simulink model "BilateralFilterHDLExample"  (R2019b)
settings: Solver=FixedStepDiscrete  StartTime=0.0  StopTime=9  RelTol=1e-3
undefined symbols (not defined in the file): gray, Rec, SDTV
libraries: visionhdlio x2, dspvision x1, visionhdlutilities x1, visionhdlfilter x1, visionhdlconversions x1, visionhdlanalysis x1
settings Model: DataTypeOverride=Off  SimulationMode=accelerator  Creator=The MathWorks, Inc.  LastModifiedBy=Bilal
settings SolverCC: MinimalZcImpactIntegration=on
settings DataIOCC: SaveOutput=off  SaveTime=off  ReturnWorkspaceOutputs=off
settings OptimizationCC: BlockReduction=off  ConditionallyExecuteInputs=off  DefaultParameterBehavior=Inlined
settings DebuggingCC: AlgebraicLoopMsg=error  SingleTaskRateTransMsg=error  ArithmeticOperatorsInVariantConditions=warning
settings HardwareCC: ProdBitPerPointer=32  ProdBitPerSizeT=32  ProdBitPerPtrDiffT=32  ProdLargestAtomicFloat=None  ProdIntDivRoundTo=Undefined  ProdEndianess=Unspecified  ProdWordSize=32  ProdHWDeviceType=ASIC/FPGA->ASIC/FPGA  ProdEqTarget=off
settings SFSimCC: SimUseLocalCustomCode=off  CustomCodeUndefinedFunction=UseInterfaceOnly
settings RTWCC: RTWUseLocalCustomCode=off
settings CodeAppCC: StateflowObjectComments=on

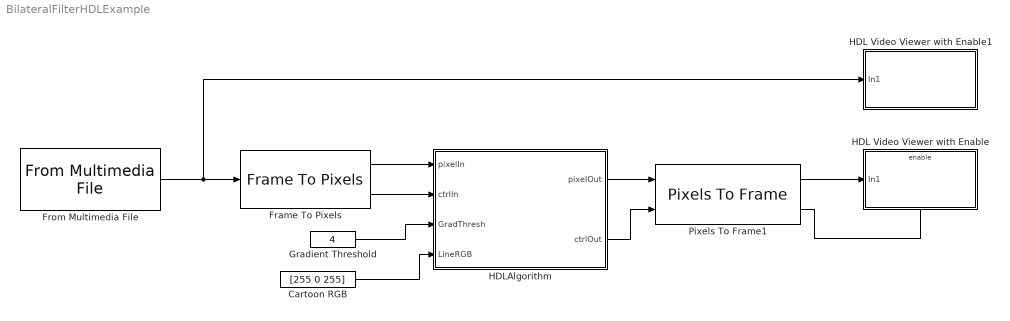
== system BilateralFilterHDLExample ==
  Cartoon RGB : Constant  Value=[255 0 255]  OutDataTypeStr=Inherit: Inherit via back propagation  SampleTime=-1
  Frame To Pixels : visionhdlio/Frame To Pixels  NumComponents=3  NumPixels=1  VideoFormat=Custom  ActivePixelsPerLine=320  ActiveVideoLines=180  TotalPixelsPerLine=400  TotalVideoLines=240  StartingActiveLine=6  FrontPorch=10  SampleTime=0
      settings: SourceProductName=Vision HDL Toolbox  SourceProductBaseCode=VT
  From Multimedia File : dspvision/From Multimedia File  inputFilename=potholes2.avi  readRange=[1 Inf]  loop=on  numPlays=inf  outputStreams=Video only  videoDataType=uint8  audioDataType=int16  inheritSampleTime=on  userDefinedSampleTime=1/30  noAudioOutput=off  isIntensityVideo=off  fourcc=RGB  colorVideoFormat=One multidimensional signal  outputEOF=off  dataOrg=Column-major  audioFrameSize=1024  computeAudioFrameSize=off  outSamplingMode=Sample based
      settings: SourceProductName=DSP System Toolbox  SourceProductBaseCode=DS
  Gradient Threshold : Constant  Value=4  OutDataTypeStr=uint8  SampleTime=-1
  HDL Video Viewer with Enable : Subsystem
  HDL Video Viewer with Enable1 : Subsystem
  HDLAlgorithm : Subsystem
  Pixels To Frame1 : visionhdlio/Pixels To Frame  NumComponents=3  NumPixels=1  VideoFormat=Custom  ActivePixelsPerLine=320  ActiveVideoLines=180  TotalPixelsPerLine=400  TotalVideoLines=240
      settings: SourceProductName=Vision HDL Toolbox  SourceProductBaseCode=VT
  wires:
  Frame To Pixels/1 -> HDLAlgorithm/1(pixelIn)
  HDLAlgorithm/2(ctrlOut) -> Pixels To Frame1/2
  HDLAlgorithm/1(pixelOut) -> Pixels To Frame1/1
  Frame To Pixels/2 -> HDLAlgorithm/2(ctrlIn)
  Pixels To Frame1/1 -> HDL Video Viewer with Enable/1(In1)
  Pixels To Frame1/2 -> HDL Video Viewer with Enable/Enable
  From Multimedia File/1 -> HDL Video Viewer with Enable1/1(In1), Frame To Pixels/1
  Gradient Threshold/1 -> HDLAlgorithm/3(GradThresh)
  Cartoon RGB/1 -> HDLAlgorithm/4(LineRGB)

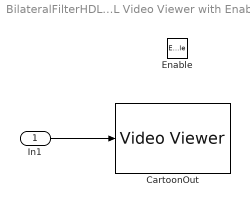
== system BilateralFilterHDLExample/HDL Video Viewer with Enable ==
  In1 : Inport
  Enable : EnablePort
  CartoonOut : VideoViewer  colormapValue=gray(256)  FigPos=[420 351 320 243]
  wires:
  In1/1 -> CartoonOut/1

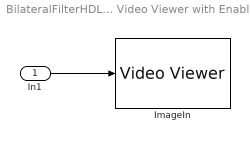
== system BilateralFilterHDLExample/HDL Video Viewer with Enable1 ==
  In1 : Inport
  ImageIn : VideoViewer  colormapValue=gray(256)  FigPos=[249 353 321 244]
  wires:
  In1/1 -> ImageIn/1

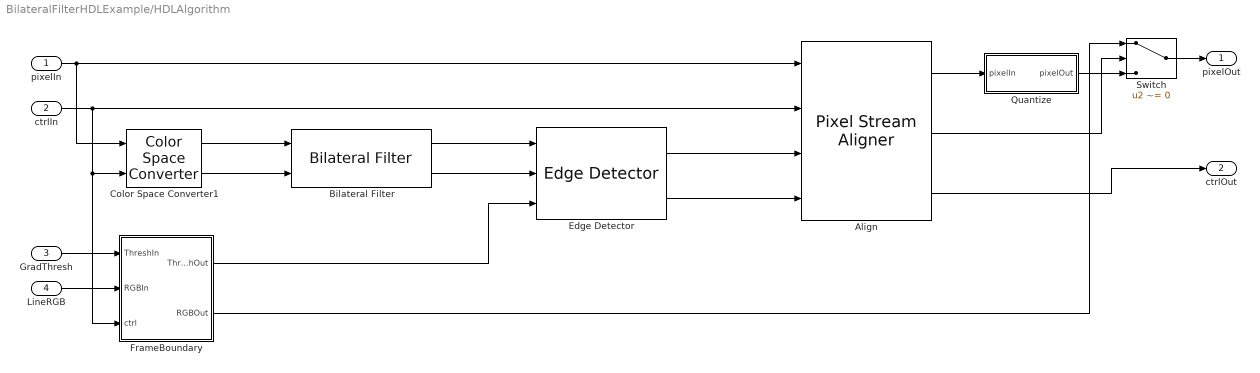
== system BilateralFilterHDLExample/HDLAlgorithm ==
  pixelIn : Inport
  ctrlIn : Inport  Port=2
  GradThresh : Inport  Port=3
  LineRGB : Inport  Port=4
  Align : visionhdlutilities/Pixel Stream Aligner  LineBufferSize=2048  MaximumNumberOfLines=10  SimulateUsing=Code generation
      settings: SourceProductName=Vision HDL Toolbox  SourceProductBaseCode=VT
  Bilateral Filter : visionhdlfilter/Bilateral Filter  NeighborhoodSize=9x9  SpatialStdDev=3  IntensityStdDev=0.75  PaddingMethod=Replicate  PaddingValue=0  LineBufferSize=2048  SimulateUsing=Code generation  CoefficientsDataTypeStr=fixdt(0,22,22)  roundingMode=Nearest  overflowMode=on  OutputDataTypeStr=fixdt(0,8,0)  OutputMin=[]  OutputMax=[]
      settings: SourceProductName=Vision HDL Toolbox  SourceProductBaseCode=VT
  Color Space Converter1 : visionhdlconversions/Color Space Converter  Conversion=RGB to intensity  ConversionStandard=Rec. 601 (SDTV)  ScanningStandard=1250/50/2:1  SimulateUsing=Code generation
      settings: SourceProductName=Vision HDL Toolbox  SourceProductBaseCode=VT
  Edge Detector : visionhdlanalysis/Edge Detector  Method=Sobel  BinaryImageOutputPort=on  GradientComponentOutputPorts=off  ThresholdSource=Input port  Threshold=20  LineBufferSize=2048  SimulateUsing=Code generation  roundingMode=Floor  overflowMode=off  GradientMin=[]  GradientMax=[]
      settings: SourceProductName=Vision HDL Toolbox  SourceProductBaseCode=VT
  FrameBoundary : Subsystem
  Quantize : Subsystem
  Switch : Switch  Criteria=u2 ~= 0
  pixelOut : Outport  VectorParamsAs1DForOutWhenUnconnected=off
  ctrlOut : Outport  Port=2  VectorParamsAs1DForOutWhenUnconnected=off
  wires:
  Color Space Converter1/2 -> Bilateral Filter/2
  ctrlIn/1 -> FrameBoundary/3(ctrl), Color Space Converter1/2, Align/2
  pixelIn/1 -> Color Space Converter1/1, Align/1
  Color Space Converter1/1 -> Bilateral Filter/1
  Align/1 -> Quantize/1(pixelIn)
  GradThresh/1 -> FrameBoundary/1(ThreshIn)
  LineRGB/1 -> FrameBoundary/2(RGBIn)
  FrameBoundary/1(ThreshOut) -> Edge Detector/3
  Align/3 -> ctrlOut/1
  Bilateral Filter/1 -> Edge Detector/1
  Bilateral Filter/2 -> Edge Detector/2
  Edge Detector/2 -> Align/4
  Edge Detector/1 -> Align/3
  Switch/1 -> pixelOut/1
  Quantize/1(pixelOut) -> Switch/3
  Align/2 -> Switch/2
  FrameBoundary/2(RGBOut) -> Switch/1

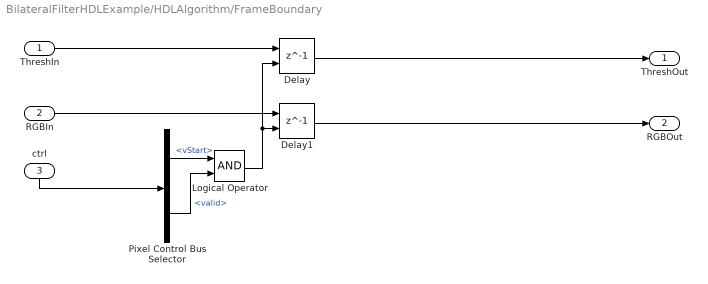
== system BilateralFilterHDLExample/HDLAlgorithm/FrameBoundary ==
  ThreshIn : Inport
  RGBIn : Inport  Port=2
  ctrl : Inport  Port=3
  Delay : Delay  DelayLength=1  ShowEnablePort=on
      settings: InputPortMap=u0,e6
  Delay1 : Delay  DelayLength=1  ShowEnablePort=on
      settings: InputPortMap=u0,e6
  Logical Operator : Logic  AllPortsSameDT=off  OutDataTypeStr=boolean
  Pixel Control Bus Selector : BusSelector  OutputSignals=vStart,valid
  ThreshOut : Outport  VectorParamsAs1DForOutWhenUnconnected=off
  RGBOut : Outport  Port=2  VectorParamsAs1DForOutWhenUnconnected=off
  wires:
  ctrl/1 -> Pixel Control Bus Selector/1
  Pixel Control Bus Selector/1 -> Logical Operator/1  "<vStart>"
  ThreshIn/1 -> Delay/1
  Logical Operator/1 -> Delay1/2, Delay/2
  Pixel Control Bus Selector/2 -> Logical Operator/2  "<valid>"
  Delay1/1 -> RGBOut/1
  RGBIn/1 -> Delay1/1
  Delay/1 -> ThreshOut/1

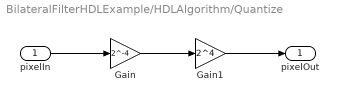
== system BilateralFilterHDLExample/HDLAlgorithm/Quantize ==
  pixelIn : Inport
  Gain : Gain  Gain=2^-4  OutDataTypeStr=Inherit: Same as input
  Gain1 : Gain  Gain=2^4  OutDataTypeStr=Inherit: Same as input
  pixelOut : Outport  VectorParamsAs1DForOutWhenUnconnected=off
  wires:
  Gain1/1 -> pixelOut/1
  Gain/1 -> Gain1/1
  pixelIn/1 -> Gain/1
